simulink model "vehicle_model_skeleton_train"  (R2014a)
settings: Solver=ode45  StartTime=0.0  StopTime=10  FixedStep=0.01  MaxStep=0.001  RelTol=1e-3
settings Model: Creator=igo  LastModifiedBy=berlinmac
settings DataIOCC: SignalLoggingSaveFormat=ModelDataLogs
settings OptimizationCC: ExpressionDepthLimit=2147483647
settings DebuggingCC: UnderspecifiedInitializationDetection=Classic  FcnCallInpInsideContextMsg=UseLocalSettings  StateNameClashWarn=warning
settings SFSimCC: SimParseCustomCode=off
settings GRTTargetCC: CombineOutputUpdateFcns=off  GRTInterface=on

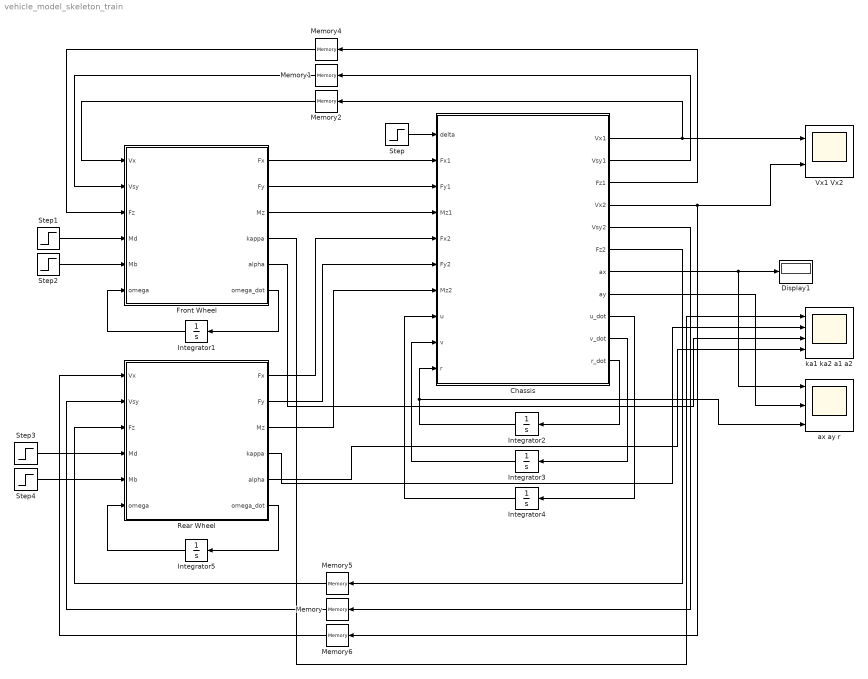
== system vehicle_model_skeleton_train ==
  Chassis : MATLAB Function  TreatAsAtomicUnit=on
  Display1 : Display
  Front Wheel : MATLAB Function  TreatAsAtomicUnit=on
  Integrator1 : Integrator  InitialCondition=66.67
  Integrator2 : Integrator
  Integrator3 : Integrator
  Integrator4 : Integrator  InitialCondition=20
  Integrator5 : Integrator  InitialCondition=66.67
  Memory : Memory
  Memory1 : Memory
  Memory2 : Memory  X0=20
  Memory4 : Memory  X0=(1500*9.8)/2
  Memory5 : Memory  X0=(1500*9.8)/2
  Memory6 : Memory  X0=20
  Rear Wheel : MATLAB Function  TreatAsAtomicUnit=on
  Step : Step  After=0.02  SampleTime=0
  Step{1..4} (4 alike) : Step  Time=0  After=0  SampleTime=0
  Vx1 Vx2 : Scope  NumInputPorts=2
      settings: TickLabels=on  ShowLegends=on  YMin=-5~-5  YMax=5~5  SaveName=ax2
  "ax ay r " : Scope  NumInputPorts=3
      settings: TickLabels=on  ShowLegends=on  TimeRange=2  YMin=-5~-5~-5  YMax=5~5~5  SaveName=ax1
  "ka1 ka2 a1 a2 " : Scope  NumInputPorts=4
      settings: TickLabels=on  ShowLegends=on  TimeRange=2  YMin=8.8e-06~8.8e-06~-0.016725~-0.0162  YMax=8.975e-06~8.975e-06~-0.016575~-0.01605  SaveName=ax
  wires:
  Front Wheel/1(Fx) -> Chassis/2(Fx1)
  Step/1 -> Chassis/1(delta)
  Chassis/11(r_dot) -> Integrator2/1
  Integrator2/1 -> Chassis/10(r), "ax ay r "/3
  Chassis/10(v_dot) -> Integrator3/1
  Integrator3/1 -> Chassis/9(v)
  Chassis/9(u_dot) -> Integrator4/1
  Integrator4/1 -> Chassis/8(u)
  Chassis/2(Vsy1) -> Memory1/1
  Chassis/5(Vsy2) -> Memory/1
  Chassis/1(Vx1) -> Vx1 Vx2/1, Memory2/1
  Memory2/1 -> Front Wheel/1(Vx)
  Memory1/1 -> Front Wheel/2(Vsy)
  Chassis/3(Fz1) -> Memory4/1
  Memory4/1 -> Front Wheel/3(Fz)
  Rear Wheel/1(Fx) -> Chassis/5(Fx2)
  Rear Wheel/2(Fy) -> Chassis/6(Fy2)
  Memory/1 -> Rear Wheel/2(Vsy)
  Chassis/4(Vx2) -> Vx1 Vx2/2, Memory6/1
  Memory6/1 -> Rear Wheel/1(Vx)
  Memory5/1 -> Rear Wheel/3(Fz)
  Chassis/6(Fz2) -> Memory5/1
  Front Wheel/6(omega_dot) -> Integrator1/1
  Integrator1/1 -> Front Wheel/6(omega)
  Rear Wheel/6(omega_dot) -> Integrator5/1
  Integrator5/1 -> Rear Wheel/6(omega)
  Front Wheel/2(Fy) -> Chassis/3(Fy1)
  Front Wheel/3(Mz) -> Chassis/4(Mz1)
  Rear Wheel/3(Mz) -> Chassis/7(Mz2)
  Step4/1 -> Rear Wheel/5(Mb)
  Step3/1 -> Rear Wheel/4(Md)
  Step1/1 -> Front Wheel/4(Md)
  Step2/1 -> Front Wheel/5(Mb)
  Chassis/7(ax) -> "ax ay r "/1, Display1/1
  Front Wheel/4(kappa) -> "ka1 ka2 a1 a2 "/1
  Rear Wheel/4(kappa) -> "ka1 ka2 a1 a2 "/2
  Front Wheel/5(alpha) -> "ka1 ka2 a1 a2 "/3
  Rear Wheel/5(alpha) -> "ka1 ka2 a1 a2 "/4
  Chassis/8(ay) -> "ax ay r "/2

== matlab function vehicle_model_skeleton_train/Front Wheel ==
  data: Vx input; Fx output; Vsy input; Fz input; Md input; Mb input; Fy output; Mz output; kappa output; alpha output; omega input; omega_dot output
function [Fx,Fy,Mz,kappa,alpha,omega_dot]=brush_tyre(Vx,Vsy,Fz,Md,Mb,omega)

%apply the brush model but not the magic formula
rf=0.3;
cp=9e6;
mu=1.2;
cz=250000;
Ip=2;
eps=0; %% to avoid the deadlock

rho=max(0,Fz/cz);
r=rf;%%only in this place, the tyre will be rigid
a=0.35*rf*(rho/rf+2.25*sqrt(rho/rf));%% P126 Empirical formula

Vr=omega*rf;
Vsx=Vx-Vr;

sigmax=-Vsx/abs(Vr);
sigmay=-Vsy/abs(Vr);
sigma=sqrt(sigmax^2+sigmay^2+eps);

alpha= -atan2(-Vsy,Vx);
kappa=-Vsx/abs(Vx+eps);

Theta=2*cp*a^2/(3*mu*Fz+eps); 
sigmasl=1/Theta;

  if sigma< sigmasl
    F=mu*Fz*Theta*sigma*(3-3*abs(Theta*sigma)+(Theta*sigma)^2); 
    t=1/3*a*(1-3*abs(Theta*sigma)+3*abs(Theta*sigma)^2-abs(Theta*sigma)^3)/(1-abs(Theta*sigma)+1/3*abs(Theta*sigma)^2);
    
        else
        F=mu*Fz;
        t=0;   
  end
         
    Fx=F*sigmax/sigma;
    Fy=F*sigmay/sigma;
    Mz=-t*Fy;
    
    
omega_dot=(-Fx*r+Md-Mb)/Ip;

return

== matlab function vehicle_model_skeleton_train/Rear Wheel ==
  data: Vx input; Fx output; Vsy input; Fz input; Md input; Mb input; Fy output; Mz output; kappa output; alpha output; omega input; omega_dot output
function [Fx,Fy,Mz,kappa,alpha,omega_dot]=brush_tyre(Vx,Vsy,Fz,Md,Mb,omega)
%apply the brush model but not the magic formula
rf=0.3;
cp=9e6;
mu=1.2;
cz=250000;
Ip=2;
eps=0;

rho=max(0,Fz/cz);
r=rf;%%only in this place, the tyre will be rigid
a=0.35*rf*(rho/rf+2.25*sqrt(rho/rf));%% P126 Empirical formula

Vr=omega*rf;
Vsx=Vx-Vr;

sigmax=-Vsx/abs(Vr);
sigmay=-Vsy/abs(Vr);
sigma=sqrt(sigmax^2+sigmay^2+eps);

alpha= -atan2(-Vsy,Vx);
kappa=-Vsx/abs(Vx+eps);

Theta=2*cp*a^2/(3*mu*Fz+eps); 
sigmasl=1/Theta;

  if sigma< sigmasl
    F=mu*Fz*Theta*sigma*(3-3*abs(Theta*sigma)+(Theta*sigma)^2); 
    t=1/3*a*(1-3*abs(Theta*sigma)+3*abs(Theta*sigma)^2-abs(Theta*sigma)^3)/(1-abs(Theta*sigma)+1/3*abs(Theta*sigma)^2);
        else
        F=mu*Fz;
        t=0;   
  end
  
   Fx=F*sigmax/sigma;
    Fy=F*sigmay/sigma;
    Mz=-t*Fy
    
    
omega_dot=(-Fx*r+Md-Mb)/Ip;

return

== matlab function vehicle_model_skeleton_train/Chassis ==
  data: delta input; Fx1 input; Fy1 input; Mz1 input; Fx2 input; Fy2 input; Mz2 input; u input; Vx1 output; v input; r input; Vsy1 output; Fz1 output; Vx2 output; Vsy2 output; Fz2 output; ax output; ay output; u_dot output; v_dot output; r_dot output

function [Vx1,Vsy1,Fz1,Vx2,Vsy2,Fz2,ax,ay,u_dot,v_dot,r_dot] = chassis_dynamics(delta,Fx1,Fy1,Mz1,Fx2,Fy2,Mz2,u,v,r)
%the right turning is positive
%1 for front Axle and 2 for rear Axle
%Fx Fy Mz from Tyre Model
a=1.5;
l=3;% wheel base
b=l-a;
Izz=2700;
m=1500;
h=0.6;
g=9.8;

u1=u;
u2=u;
v1=v+a*r;
v2=v-b*r;

Vx1=u1*cos(delta)+v1*sin(delta);
Vsy1=-u1*sin(delta)+v1*cos(delta);

Vx2=u2;
Vsy2=v2;

Fx1c=Fx1*cos(delta)-Fy1*sin(delta);
Fy1c=Fx1*sin(delta)+Fy1*cos(delta);

Fx2c=Fx2;
Fy2c=Fy2;

Fxc=Fx1c+Fx2c;
Fyc=Fy1c+Fy2c;
Mz=Fy1c.*a+Mz1-Fy2c.*b+Mz2;

deltaFz=h./l*Fxc;

Fz1=b/l*m*g-deltaFz;
Fz2=a/l*m*g+deltaFz;

ax=Fxc./m;
ay=Fyc./m;

u_dot=ax+v*r; 
v_dot=ay-u*r;
r_dot=Mz/Izz;


return
